simulink model "Regelungslabor_02_Aufgabe_02_b_schaltung"  (R2023b)
settings: Solver=VariableStepAuto  StartTime=0.0  StopTime=10.0  RelTol=1e-3
values from neighbouring files (symbols this model uses):
  AB = 0.0226    [Reglungslabor_02_Aufgabe_2_b_skript.m]
  c = 0.003    [Reglungslabor_02_Aufgabe_2_b_skript.m]
  h = 0.1    [Reglungslabor_02_Aufgabe_2_b_skript.m]
  KR = 0.01    [Reglungslabor_02_Aufgabe_2_b_skript.m]
  sim_time = 70    [Reglungslabor_02_Aufgabe_2_b_skript.m]
  TN = TN_array(count)    [Reglungslabor_02_Aufgabe_2_b_skript.m]
settings Model: Creator=danie  LastModifiedBy=danie

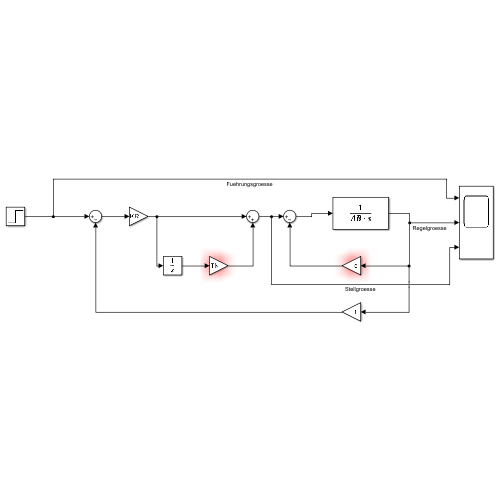
[thumbnail: Simulink's stored preview of the top-level diagram]
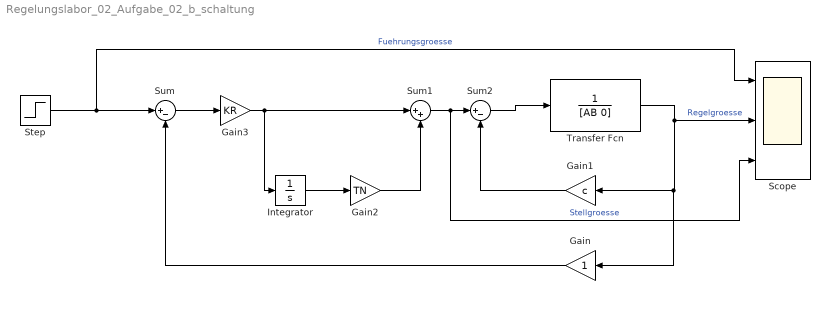
== system Regelungslabor_02_Aufgabe_02_b_schaltung ==
  Gain : Gain
  Gain1 : Gain  Gain=c
  Gain2 : Gain  Gain=TN
  Gain3 : Gain  Gain=KR
  Integrator : Integrator
  Scope : Scope  NumInputPorts=3
  Step : Step  Time=sim_time  Before=h  SampleTime=0
  Sum : Sum  Inputs=|+-
  Sum1 : Sum  Inputs=|++
  Sum2 : Sum  Inputs=|+-
  Transfer Fcn : TransferFcn  Denominator=[AB 0]
  wires:
  Sum/1 -> Gain3/1
  Gain3/1 -> Integrator/1, Sum1/1
  Sum2/1 -> Transfer Fcn/1
  Transfer Fcn/1 -> Scope/2, Gain/1, Gain1/1  "Regelgroesse"
  Gain1/1 -> Sum2/2
  Integrator/1 -> Gain2/1
  Gain2/1 -> Sum1/2
  Gain/1 -> Sum/2
  Step/1 -> Scope/1, Sum/1  "Fuehrungsgroesse"
  Sum1/1 -> Scope/3, Sum2/1  "Stellgroesse"
